simulink model "ARI_16_PozorovatelKyvadlo"  (Simulink 8.0)
settings: Solver=ode45  StartTime=0.0  StopTime=1  RelTol=1e-3
settings Model: Creator=Michael  ModifiedByFormat=Michael Sebek  LastModifiedBy=Michael Sebek
settings DataIOCC: SignalLoggingSaveFormat=ModelDataLogs
settings OptimizationCC: InitFltsAndDblsToZero=on
settings DebuggingCC: SaveWithParameterizedLinksMsg=none  SignalResolutionControl=TryResolveAllWithWarning  MultiTaskDSMMsg=warning  MultiTaskCondExecSysMsg=none  FcnCallInpInsideContextMsg=UseLocalSettings  StrictBusMsg=None
settings RTWCC: IncludeERTFirstTime=on
settings GRTTargetCC: TargetFcnLib=ansi_tfl_tmw.mat  CombineOutputUpdateFcns=off  GRTInterface=on

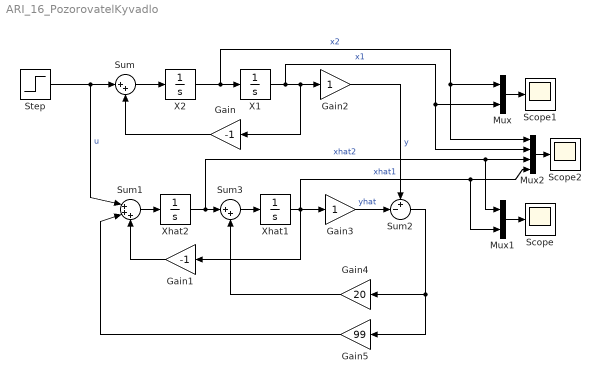
== system ARI_16_PozorovatelKyvadlo ==
  Gain : Gain  Gain=-1
  Gain1 : Gain  Gain=-1
  Gain2 : Gain
  Gain3 : Gain
  Gain4 : Gain  Gain=20
  Gain5 : Gain  Gain=99
  Mux : Mux  Inputs=2
  Mux1 : Mux  Inputs=2
  Mux2 : Mux
  Scope : Scope
  Scope1 : Scope
  Scope2 : Scope
      settings: SaveName=ScopeData2
  Step : Step  SampleTime=0
  Sum : Sum  Inputs=|++
  Sum1 : Sum  Inputs=|+++
  Sum2 : Sum  Inputs=+-|
  Sum3 : Sum  Inputs=|++
  X1 : Integrator  InitialCondition=-1
  X2 : Integrator  InitialCondition=3
  Xhat1 : Integrator
  Xhat2 : Integrator
  wires:
  X2/1 -> X1/1, Mux/1, Mux2/1  "x2"
  Sum/1 -> X2/1
  Step/1 -> Sum/1, Sum1/1  "u"
  Gain/1 -> Sum/2
  X1/1 -> Gain/1, Gain2/1, Mux/2, Mux2/2  "x1"
  Sum1/1 -> Xhat2/1
  Xhat1/1 -> Gain1/1, Gain3/1, Mux1/2, Mux2/4  "xhat1"
  Gain2/1 -> Sum2/1  "y"
  Gain3/1 -> Sum2/2  "yhat"
  Xhat2/1 -> Mux1/1, Mux2/3, Sum3/1  "xhat2"
  Sum3/1 -> Xhat1/1
  Gain4/1 -> Sum3/2
  Gain5/1 -> Sum1/2
  Gain1/1 -> Sum1/3
  Sum2/1 -> Gain4/1, Gain5/1
  Mux1/1 -> Scope/1
  Mux/1 -> Scope1/1
  Mux2/1 -> Scope2/1
